simulink model "mission"  (R2018b)
settings: Solver=VariableStepAuto  StartTime=0.0  StopTime=500  RelTol=1e-3
settings Model: Creator=miguel  LastModifiedBy=miguel
settings SFSimCC: SimUseLocalCustomCode=off
settings RTWCC: RTWUseLocalCustomCode=off

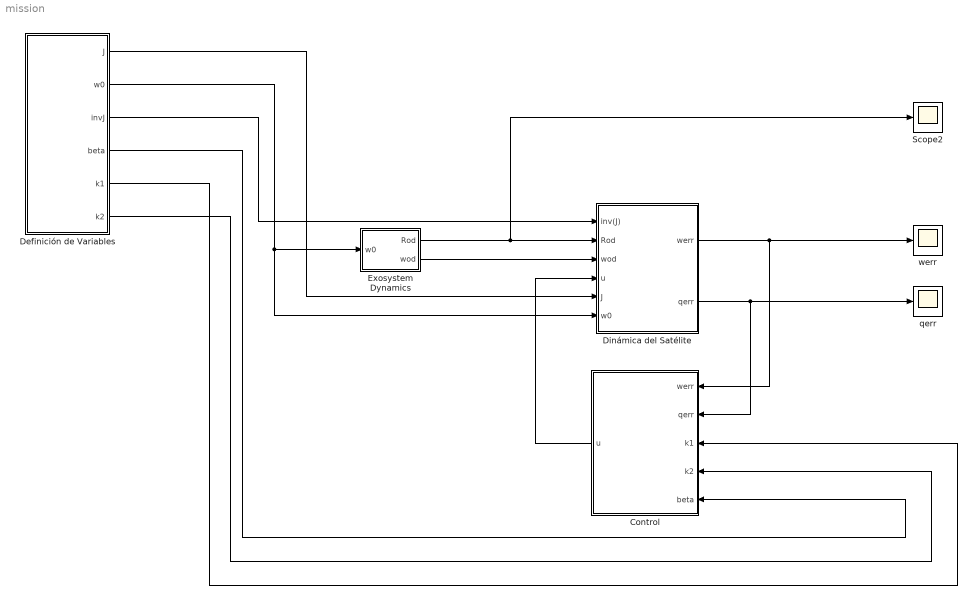
== system mission ==
  Control : Subsystem
  Definición de Variables : MATLAB Function  TreatAsAtomicUnit=on
  Dinámica del Satélite : Subsystem
  "Exosystem Dynamics " : Subsystem
  Scope2 : Scope
  qerr : Scope
  werr : Scope
  wires:
  Control/1(u) -> Dinámica del Satélite/4(u)
  Dinámica del Satélite/1(werr) -> Control/1(werr), werr/1
  Dinámica del Satélite/2(qerr) -> qerr/1, Control/2(qerr)
  "Exosystem Dynamics "/1(Rod) -> Scope2/1, Dinámica del Satélite/2(Rod)
  "Exosystem Dynamics "/2(wod) -> Dinámica del Satélite/3(wod)
  Definición de Variables/6(k2) -> Control/4("k2 ")
  Definición de Variables/2(w0) -> Dinámica del Satélite/6(w0), "Exosystem Dynamics "/1(w0)
  Definición de Variables/5(k1) -> Control/3(k1)
  Definición de Variables/3(invJ) -> Dinámica del Satélite/1("inv(J) ")
  Definición de Variables/4(beta) -> Control/5(beta)
  Definición de Variables/1(J) -> Dinámica del Satélite/5(J)

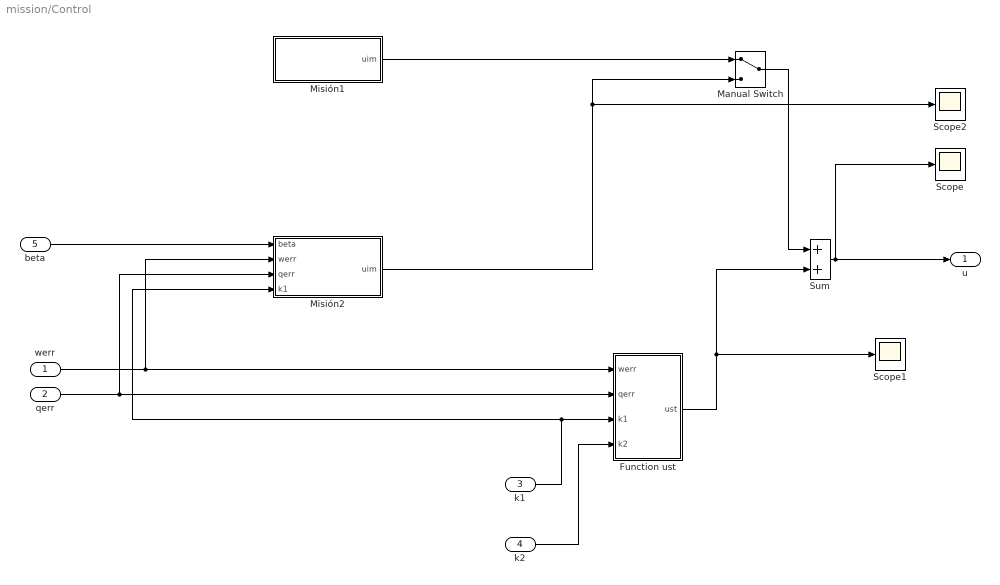
== system mission/Control ==
  werr : Inport
  qerr : Inport  Port=2
  k1 : Inport  Port=3
  "k2 " : Inport  Port=4
  beta : Inport  Port=5
  Function ust : MATLAB Function  TreatAsAtomicUnit=on
  Manual Switch : ManualSwitch
  "Misión1 " : Subsystem
  Misión2 : Subsystem
  Scope : Scope
  Scope1 : Scope
  Scope2 : Scope
  Sum : Sum
  u : Outport
  wires:
  Sum/1 -> Scope/1, u/1
  qerr/1 -> Misión2/3(qerr), Function ust/2(qerr)
  werr/1 -> Misión2/2(werr), Function ust/1(werr)
  k1/1 -> Function ust/3(k1), Misión2/4(k1)
  "k2 "/1 -> Function ust/4(k2)
  Function ust/1(ust) -> Scope1/1, Sum/2
  "Misión1 "/1(uim) -> Manual Switch/1
  Manual Switch/1 -> Sum/1
  Misión2/1(uim) -> Scope2/1, Manual Switch/2
  beta/1 -> Misión2/1(beta)

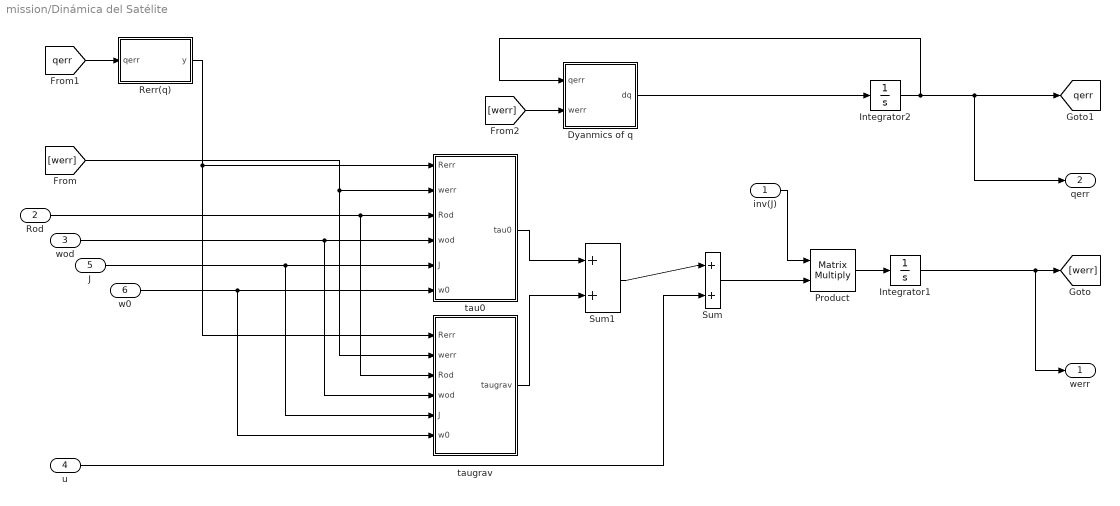
== system mission/Dinámica del Satélite ==
  "inv(J) " : Inport
  Rod : Inport  Port=2
  wod : Inport  Port=3
  u : Inport  Port=4
  J : Inport  Port=5
  w0 : Inport  Port=6
  Dyanmics of q : MATLAB Function  TreatAsAtomicUnit=on
  Integrator1 : Integrator  InitialCondition=[0;6.2*10^-3;0]
  Integrator2 : Integrator  InitialCondition=[0.968;-0.2;-0.1;0.1]
  Product : Product  Multiplication=Matrix(*)
  Rerr(q) : MATLAB Function  TreatAsAtomicUnit=on
  Sum : Sum  Inputs=|++
  Sum1 : Sum
  tau0 : MATLAB Function  TreatAsAtomicUnit=on
  taugrav : MATLAB Function  TreatAsAtomicUnit=on
  werr : Outport
  qerr : Outport  Port=2
  tag scope: qerr=global
  wires:
  Dyanmics of q/1(dq) -> Integrator2/1
  Product/1 -> Integrator1/1
  Sum/1 -> Product/2
  Integrator1/1 -> [werr], werr/1
  u/1 -> Sum/2
  "inv(J) "/1 -> Product/1
  Integrator2/1 -> Dyanmics of q/1(qerr), qerr/1, [qerr]
  Rerr(q)/1(y) -> taugrav/1(Rerr), tau0/1(Rerr)
  tau0/1(tau0) -> Sum1/1
  taugrav/1(taugrav) -> Sum1/2
  Sum1/1 -> Sum/1
  wod/1 -> taugrav/4(wod), tau0/4(wod)
  Rod/1 -> taugrav/3(Rod), tau0/3(Rod)
  [werr] -> taugrav/2(werr), tau0/2(werr)
  [qerr] -> Rerr(q)/1(qerr)
  [werr] -> Dyanmics of q/2(werr)
  J/1 -> taugrav/5(J), tau0/5(J)
  w0/1 -> taugrav/6(w0), tau0/6(w0)

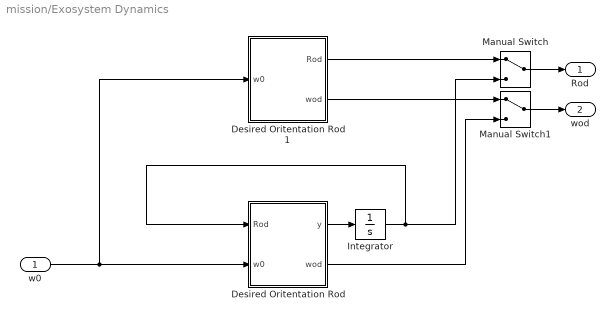
== system mission/Exosystem Dynamics  ==
  w0 : Inport
  "Desired Oritentation Rod " : MATLAB Function  TreatAsAtomicUnit=on
  Desired Oritentation Rod 1 : MATLAB Function  TreatAsAtomicUnit=on
  Integrator : Integrator  InitialCondition=[1 0 0;0 1 0;0 0 1]
  Manual Switch : ManualSwitch
  Manual Switch1 : ManualSwitch
  Rod : Outport
  wod : Outport  Port=2
  wires:
  Integrator/1 -> Manual Switch/2, "Desired Oritentation Rod "/1(Rod)
  "Desired Oritentation Rod "/1(y) -> Integrator/1
  "Desired Oritentation Rod "/2(wod) -> Manual Switch1/2
  w0/1 -> Desired Oritentation Rod 1/1(w0), "Desired Oritentation Rod "/2(w0)
  Desired Oritentation Rod 1/1(Rod) -> Manual Switch/1
  Desired Oritentation Rod 1/2(wod) -> Manual Switch1/1
  Manual Switch1/1 -> wod/1
  Manual Switch/1 -> Rod/1

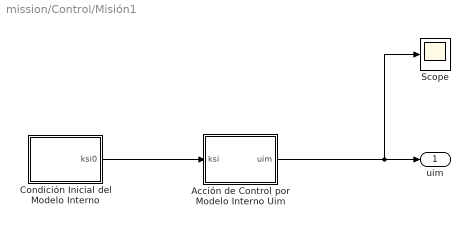
== system mission/Control/Misión1  ==
  Acción de Control por Modelo Interno Uim : MATLAB Function  TreatAsAtomicUnit=on
  Condición Inicial del Modelo Interno : MATLAB Function  TreatAsAtomicUnit=on
  Scope : Scope
  uim : Outport
  wires:
  Acción de Control por Modelo Interno Uim/1(uim) -> Scope/1, uim/1
  Condición Inicial del Modelo Interno/1(ksi0) -> Acción de Control por Modelo Interno Uim/1(ksi)

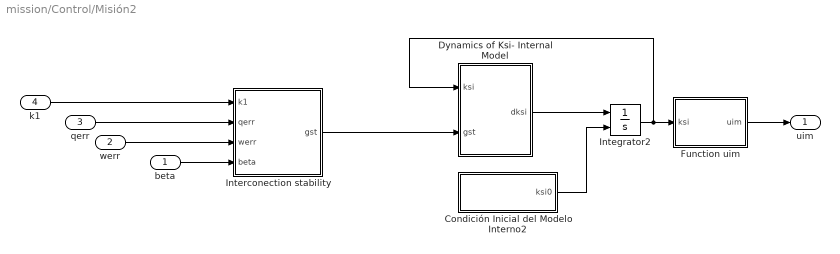
== system mission/Control/Misión2 ==
  beta : Inport
  werr : Inport  Port=2
  qerr : Inport  Port=3
  k1 : Inport  Port=4
  "Condición Inicial del Modelo Interno2 " : MATLAB Function  TreatAsAtomicUnit=on
  "Dynamics of Ksi- Internal Model " : MATLAB Function  TreatAsAtomicUnit=on
  Function uim : MATLAB Function  TreatAsAtomicUnit=on
  Integrator2 : Integrator  InitialConditionSource=external  InitialCondition=[0;0;0;0;0;0;0;0;0;0;0.3925*10^-5;0;0;0;0]
  Interconection stability : MATLAB Function  TreatAsAtomicUnit=on
  uim : Outport
  wires:
  beta/1 -> Interconection stability/4(beta)
  qerr/1 -> Interconection stability/2(qerr)
  "Condición Inicial del Modelo Interno2 "/1(ksi0) -> Integrator2/2
  "Dynamics of Ksi- Internal Model "/1(dksi) -> Integrator2/1
  k1/1 -> Interconection stability/1(k1)
  Function uim/1(uim) -> uim/1
  Interconection stability/1(gst) -> "Dynamics of Ksi- Internal Model "/2(gst)
  werr/1 -> Interconection stability/3(werr)
  Integrator2/1 -> "Dynamics of Ksi- Internal Model "/1(ksi), Function uim/1(ksi)

== matlab function mission/Exosystem Dynamics /Desired Oritentation Rod  ==
  data: Rod input; y output; w0 input; wod output
function [y, wod] = fcn(Rod,w0)

wod=[0;w0;0];

y = Rod*[0 -wod(3) wod(2);
wod(3) 0 -wod(1);
-wod(2) wod(1) 0;];

== matlab function mission/Dinámica del Satélite/Dyanmics of q ==
  data: qerr input; dq output; werr input
function dq = fcn(qerr,werr)

E=[-qerr(2) -qerr(3) -qerr(4);
qerr(1) -qerr(4) qerr(3);
qerr(4) qerr(1) -qerr(2);
-qerr(3) qerr(2) qerr(1);]

y=0.5*E*werr;

dq = y;

== matlab function mission/Control/Misión2/Dynamics of Ksi- Internal Model  ==
  data: ksi input; dksi output; gst input
function dksi = fcn(ksi, gst)

W= 6.2*10^-3; %||w(0)|| modulo de la velocidad deseada


S=[0 1 0 0 0;
0 0 1 0 0;
0 0 0 1 0;
0 0 0 0 1;
0 -4*W^4 0 -5*W^2 0];

phi=[S zeros(5,5) zeros(5,5);
zeros(5,5) S zeros(5,5);
zeros(5,5) zeros(5,5) S];


dksi = phi*ksi + gst;

== matlab function mission/Control/Function ust ==
  data: werr input; ust output; qerr input; k1 input; k2 input
function ust = fcn(werr,qerr,k1,k2)


u=-k2*(1+norm(werr+k1*[qerr(2);qerr(3);qerr(4)]))*(werr+k1*[qerr(2);qerr(3);qerr(4)]);

ust = u;

== matlab function mission/Control/Misión2/Function uim ==
  data: ksi input; uim output
function uim = fcn(ksi)

Q=[1 0 0 0 0];

gamma=[Q zeros(1,5) zeros(1,5);
zeros(1,5) Q zeros(1,5);
zeros(1,5) zeros(1,5) Q];

uim = gamma*ksi;

== matlab function mission/Dinámica del Satélite/Rerr(q) ==
  data: qerr input; y output
function y = fcn(qerr)

Rerr=[1-2*qerr(3)^2-2*qerr(4)^2 2*qerr(2)*qerr(3)-2*qerr(1)*qerr(4) 2*qerr(2)*qerr(4)+2*qerr(1)*qerr(3);
2*qerr(2)*qerr(3)+2*qerr(1)*qerr(4) 1-2*qerr(2)^2-2*qerr(4)^2 2*qerr(3)*qerr(4)-2*qerr(1)*qerr(2);
2*qerr(2)*qerr(4)-2*qerr(1)*qerr(3) 2*qerr(3)*qerr(4)+2*qerr(1)*qerr(2) 1-2*qerr(2)^2-2*qerr(3)^2]



y = Rerr;

== matlab function mission/Dinámica del Satélite/tau0 ==
  data: Rerr input; tau0 output; werr input; Rod input; wod input; J input; w0 input
function tau0 = fcn(Rerr, werr, Rod, wod, J, w0)



J=[1.3 0.2 0.08;
0.2 0.9  0.09;
0.08 0.09 1.8];
%definir la matriz J
w0= 6.2*10^-3;%definir el modulo de la velocidad angular deseada

wed= Rerr'*(wod-w0*Rod'*[0;1;0]);

dwed= -cross(werr,wed) + w0*Rerr'*(cross(wod, Rod'*[0;1;0]));


u= -cross(werr,J*werr)-cross(wed,J*werr)-cross(werr,J*wed)-cross(wed,J*wed)-J*dwed;


tau0= u;

== matlab function mission/Dinámica del Satélite/taugrav ==
  data: Rerr input; taugrav output; werr input; Rod input; wod input; J input; w0 input
function taugrav = fcn(Rerr,werr,Rod,wod, J, w0)



taugrav = 3*w0^2*cross((Rod*Rerr)'*[0;0;1],J*(Rod*Rerr)'*[0;0;1]);

== matlab function mission/Definición de Variables ==
  data: J output; w0 output; invJ output; beta output; k1 output; k2 output
function [J, w0, invJ, beta, k1, k2] = fcn

%Definimos aquí los parámetros
J=[1.3 0.2 0.08;
    0.2 0.9  0.09;
    0.08 0.09 1.8];

beta=5*10^-3;

k1=0.25;

k2=25; 

w0= 6.2*10^-3;
invJ= inv(J);

== matlab function mission/Control/Misión2/Interconection stability ==
  data: k1 input; gst output; qerr input; werr input; beta input
function gst = fcn(k1, qerr, werr, beta)



Q=[1 0 0 0 0];

gamma=[Q zeros(1,5) zeros(1,5);
zeros(1,5) Q zeros(1,5);
zeros(1,5) zeros(1,5) Q];


P= [7.95147999656573,-96.0935098307059,694.778417691778,-2150.92915678928,-4867.73558815196,0,0,0,0,0,0,0,0,0,0;
    -96.0935098307059,1817.74992527759,-17243.0452447914,74694.0163632687,112765.085416469,0,0,0,0,0,0,0,0,0,0;
    694.778417691778,-17243.0452447914,204788.295295055,-1199232.40308186,-104586.913467657,0,0,0,0,0,0,0,0,0,0;
    -2150.92915678928,74694.0163632687,-1199232.40308186,10430890.3198412,-27944049.8827230,0,0,0,0,0,0,0,0,0,0;
    -4867.73558815196,112765.085416469,-104586.913467657,-27944049.8827230,536545695.418565,0,0,0,0,0,0,0,0,0,0;
    0,0,0,0,0,7.95147999648926,-96.0935098301661,694.778417690043,-2150.92915679205,-4867.73558793617,0,0,0,0,0;
    0,0,0,0,0,-96.0935098301661,1817.74992527483,-17243.0452448153,74694.0163634383,112765.085415515,0,0,0,0,0;
    0,0,0,0,0,694.778417690043,-17243.0452448153,204788.295295984,-1199232.40308876,-104586.913467497,0,0,0,0,0;
    0,0,0,0,0,-2150.92915679205,74694.0163634383,-1199232.40308876,10430890.3199229,-27944049.8829483,0,0,0,0,0;
    0,0,0,0,0,-4867.73558793617,112765.085415515,-104586.913467497,-27944049.8829483,536545695.420330,0,0,0,0,0;
    0,0,0,0,0,0,0,0,0,0,7.95147999655389,-96.0935098311681,694.778417698825,-2150.92915683269,-4867.73558806930;
    0,0,0,0,0,0,0,0,0,0,-96.0935098311681,1817.74992529368,-17243.0452450021,74694.0163645257,112765.085415410;
    0,0,0,0,0,0,0,0,0,0,694.778417698825,-17243.0452450021,204788.295297949,-1199232.40310095,-104586.913437447;
    0,0,0,0,0,0,0,0,0,0,-2150.92915683269,74694.0163645257,-1199232.40310095,10430890.3199868,-27944049.8831210;
    0,0,0,0,0,0,0,0,0,0,-4867.73558806930,112765.085415410,-104586.913437447,-27944049.8831210,536545695.418906]


gst= -(1/beta)*inv(P)*gamma'*(werr+k1*[qerr(2);qerr(3);qerr(4)]);

== matlab function mission/Exosystem Dynamics /Desired Oritentation Rod 1 ==
  data: Rod output; w0 input; wod output
function [Rod, wod] = fcn(w0)

wod=[0; 0; 0];

Rod=[1 0 0;
    0 1 0;
    0 0 1];

== matlab function mission/Control/Misión1 /Acción de Control por Modelo Interno Uim ==
  data: ksi input; uim output
function uim = fcn(ksi)


uim = ksi;

== matlab function mission/Control/Misión1 /Condición Inicial del Modelo Interno ==
  data: ksi0 output
function ksi0 = fcn 

J=[1.3 0.2 0.08;
    0.2 0.9  0.09;
    0.08 0.09 1.8];

w0= 6.2*10^-3;


tau0= -w0^2*[J(2,3);0; J(1,2)];
taugrav= 3*w0^2*[J(2,3); J(1,3);0];


ksi0= tau0 + taugrav
%ksi0 = [-0.1384;-0.0923;0.0769]*10^-4;

== matlab function mission/Control/Misión2/Condición Inicial del Modelo Interno2  ==
  data: ksi0 output
function ksi0 = fcn


ksi0 =[-0.1384;0;0;0;0;-0.0923;0;0;0;0;0.0769;0;0;0;0]*10^-4;
